simulink model "lidar_stepper_tester"  (Simulink 7.3)
settings: Solver=FixedStepDiscrete  StartTime=0.0  StopTime=inf  RelTol=1e-3
settings Model: Creator=wildcat  LastModifiedBy=wildcat
settings DebuggingCC: FcnCallInpInsideContextMsg=Enable All  StrictBusMsg=ErrorLevel1
settings SFSimCC: SimUserLibraries=phidget21
settings RTWCC: SystemTargetFile=rlnx.tlc  GenCodeOnly=on  TemplateMakefile=rlnx_ubuntu.tmf  Description=Linux Real-Time Target  ProcessScript=rlnx_make_rtw_hook
settings RTWCC: CustomInclude=|
  | /home/wesley/Desktop/libphidget-2.1.8.20140319/
  | /home/wesley/Desktop/FAUTest/TestWithNoVideo/
settings CodeAppCC: GenerateComments=off  SimulinkBlockComments=off
settings STFCustomTargetCC: ModelReferenceCompliant=off  MatFileLogging=on  SystemTargetFile=rlnx.tlc
settings GRTTargetCC: ModelReferenceCompliant=off  ParMdlRefBuildCompliant=off  CompOptLevelCompliant=off
settings CustomProperty: DataType=string  Value=-lm -ldl -lc_urg -lc_urg_connection -lc_urg_system -lphidget21
settings EnumStrPairs: String=PC

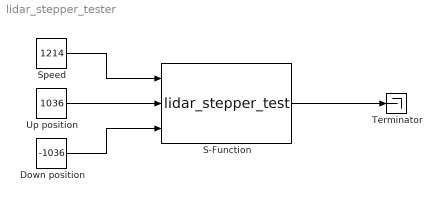
== system lidar_stepper_tester ==
  Down position : Constant  Value=-1036  OutDataType=fixdt(1, 16)  OutScaling=2^0
  S-Function : S-Function  FunctionName=lidar_stepper_test  EnableBusSupport=off
  Speed : Constant  Value=1214  OutDataType=fixdt(1, 16)  OutScaling=2^0
  Terminator : Terminator
  Up position : Constant  Value=1036  OutDataType=fixdt(1, 16)  OutScaling=2^0
  wires:
  Speed/1 -> S-Function/1
  Up position/1 -> S-Function/2
  Down position/1 -> S-Function/3
  S-Function/1 -> Terminator/1
